simulink model "host"  (R2024b)
settings: Solver=FixedStepDiscrete  StartTime=0.0  StopTime=Inf  RelTol=1e-3  EnableMultiTasking=on
InitFcn:
  | Motor_data_IM_R;
libraries: instrumentseriallib x2
settings Model: ExtModeTrigDuration=8  Creator=dario  LastModifiedBy=dario
settings OptimizationCC: DefaultParameterBehavior=Inlined  DefaultUnderspecifiedDataType=single  EnhancedBackFolding=on  PassReuseOutputArgsAs=Individual arguments  MaxStackSize=1024  OptimizeBlockOrder=speed  DifferentSizesBufferReuse=on  OptimizationCustomize=off  EfficientTunableParamExpr=on
settings DebuggingCC: ParameterTunabilityLossMsg=error
settings HardwareCC: ProdBitPerChar=16  ProdBitPerInt=16  ProdBitPerPointer=32  ProdBitPerSizeT=32  ProdBitPerPtrDiffT=32  ProdLargestAtomicInteger=Integer  ProdLargestAtomicFloat=None  ProdWordSize=16  ProdLongLongMode=on  ProdHWDeviceType=Texas Instruments->C2000  HardwareBoardFeatureSet=SoCBlockset
settings SFSimCC: MATLABDynamicMemAlloc=off
settings RTWCC: Description=Embedded Coder  SystemTargetFile=ert.tlc  HardwareBoard=TI Delfino F28379D LaunchPad  TemplateMakefile=ert_default_tmf  GenerateReport=on  Toolchain=Texas Instruments Code Composer Studio (C2000)  LaunchReport=on  CodeProfilingSaveOptions=MetricsOnly
settings CodeAppCC: ForceParamTrailComments=on  IgnoreCustomStorageClasses=off  OperatorAnnotations=on  SimulinkDataObjDesc=on  SFDataObjDesc=on  InsertBlockDesc=on
settings ERTTargetCC: CodeReplacementLibrary=TI C28x  ExtModeTransport=4  ExtModeStaticAlloc=on  ExtModeAutomaticAllocSize=off  ExtModeStaticAllocSize=10000  ExtModeMexFile=ext_xcp  ExtModeIntrfLevel=Level2 - Open

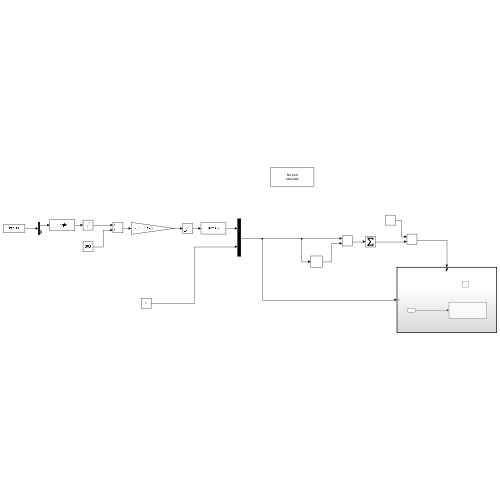
[thumbnail: Simulink's stored preview of the top-level diagram]
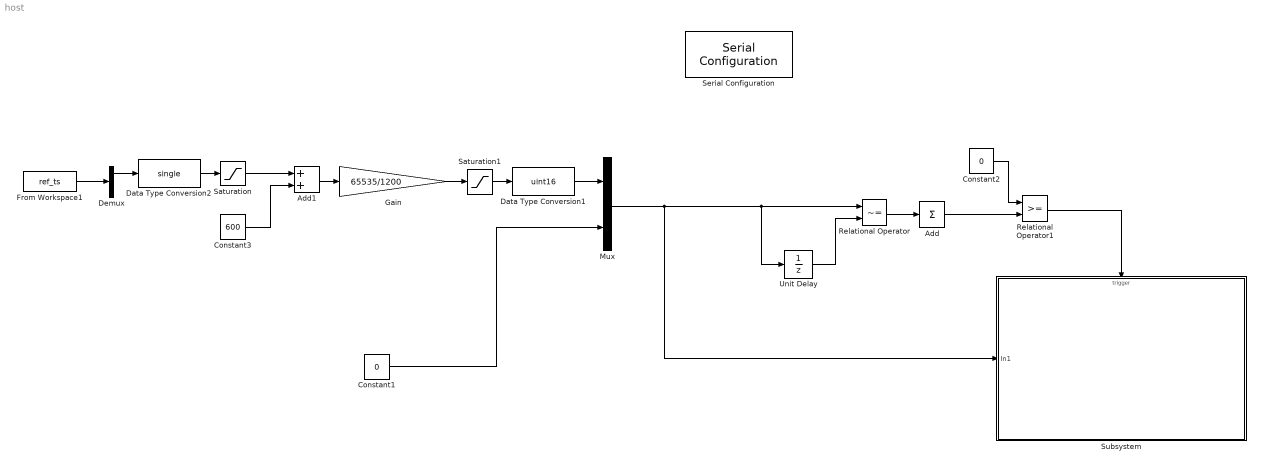
== system host ==
  Add : Sum  Inputs=+
  Add1 : Sum  OutDataTypeStr=single
  Constant1 : Constant  Value=0  OutDataTypeStr=uint16
  Constant2 : Constant  Value=0  OutDataTypeStr=uint16
  Constant3 : Constant  Value=600  OutDataTypeStr=single
  Data Type Conversion1 : DataTypeConversion  OutDataTypeStr=uint16  SaturateOnIntegerOverflow=off  RndMeth=Floor
  Data Type Conversion2 : DataTypeConversion  OutDataTypeStr=single  SaturateOnIntegerOverflow=off  RndMeth=Floor
  Demux : Demux  Outputs=2
  From Workspace1 : FromWorkspace  VariableName=ref_ts  OutDataTypeStr=single  Interpolate=off  OutputAfterFinalValue=Holding final value
  Gain : Gain  Gain=65535/1200  ParamDataTypeStr=single  OutDataTypeStr=single
  Mux : Mux  Inputs=2
  Relational Operator : RelationalOperator  Operator=~=  OutDataTypeStr=fixdt(0,16)  RndMeth=Simplest  InputSameDT=off
  Relational Operator1 : RelationalOperator  OutDataTypeStr=fixdt(0,16)  RndMeth=Simplest  InputSameDT=off
  Saturation : Saturate  UpperLimit=600  LowerLimit=-600  OutDataTypeStr=single
  Saturation1 : Saturate  UpperLimit=65535  LowerLimit=0  OutDataTypeStr=single
  Serial Configuration : instrumentseriallib/Serial Configuration  Priority=-200000  PortSel=<Select a port...>  Port=<Select a port...>  ComPort=<Select a port...>  BaudRate=5000000  DataBits=8  Parity=none  StopBits=1  ByteOrder=little-endian  FlowControl=none  Timeout=10  SimulateUsing=Interpreted execution  BlockInModel=on  aMode=1
      settings: LibrarySourceBlock=c2000lib/Host Communication/Serial Configuration
  Subsystem : Subsystem
  Unit Delay : UnitDelay  SampleTime=-1  HasFrameUpgradeWarning=on
  wires:
  Demux/1 -> Data Type Conversion2/1
  Gain/1 -> Saturation1/1
  Constant1/1 -> Mux/2
  Mux/1 -> Subsystem/1(In1), Unit Delay/1, Relational Operator/1
  Unit Delay/1 -> Relational Operator/2
  Relational Operator/1 -> Add/1
  Add/1 -> Relational Operator1/2
  Constant2/1 -> Relational Operator1/1
  Relational Operator1/1 -> Subsystem/Trigger
  From Workspace1/1 -> Demux/1
  Data Type Conversion2/1 -> Saturation/1
  Constant3/1 -> Add1/2
  Add1/1 -> Gain/1
  Saturation/1 -> Add1/1
  Saturation1/1 -> Data Type Conversion1/1
  Data Type Conversion1/1 -> Mux/1

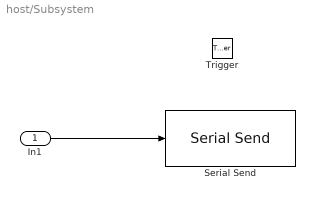
== system host/Subsystem ==
  In1 : Inport
  Trigger : TriggerPort  VariantControl=(inherit)  PortDimensions=1
  Serial Send : instrumentseriallib/Serial Send  Priority=1  PortSel=<Select a port...>  Port=<Select a port...>  ComPort=<Select a port...>  Header='SS'  Terminator=Custom terminator  CustomTerminator='EE'  EnableBlockingMode=on  SimulateUsing=Interpreted execution  BlockInModel=on  aMode=1
      settings: LibrarySourceBlock=c2000lib/Host Communication/Serial Send
  wires:
  In1/1 -> Serial Send/1
